simulink library "ddm"  (R2021b)
settings: Solver=VariableStepAuto  StartTime=0.0  StopTime=10.0  RelTol=1e-3
undefined symbols (not defined in the file or in its folder): ADDM_FrTMTqDev_X_Nm, ADDM_RrTMTqDev_X_Nm, ENUM_ADASACCSTA_ERROR, ENUM_ADASACCSTA_OFF, ENUM_ADASACCSTA_STANDBY, ENUM_ALLOWMOV_ALLOWREADY, ENUM_APS, ENUM_BRKSTA_ERROR, ENUM_BRKSTA_OFF, ENUM_BRKSTA_ON, ENUM_BRKSW_INVALID, ENUM_BRKSW_OFF, ENUM_BRKSW_ON, ENUM_CHGPREACTERRSTA_OBCPRE, ENUM_DCDCFAULTSTA_ANYFAULTLV1, ENUM_DCDCFAULTSTA_ANYFAULTLV2, ENUM_DRIVETRAIN_AWD, ENUM_DRIVETRAIN_FWD, ENUM_DRIVETRAIN_RWD, ENUM_EDUDRTSTA_NORMAL, ENUM_EPBSTA_APPLIED, ENUM_EPBSTA_RELEASED, ENUM_ESCAPSSta_APSUNAVAILABLE, ENUM_GEARACTUALPOSN_INVALID, ENUM_GEARACTUALPOSN_P, ENUM_HVBATTREADYPRE_READY, ENUM_MCUWARN_LV0, ENUM_MCUWARN_LV1, ENUM_MCUWARN_LV2, ENUM_MCUWARN_LV3, ENUM_MCUWARN_NOERROR, ENUM_OBCFAULTSTA_ANYFAULT, ENUM_PAS_R2F2, ENUM_PDFAULT_BATTPDFAIL, ENUM_PDFAULT_DCDCDISABLE, ENUM_PDFAULT_MCUDISABLE, ENUM_PDFAULT_MCUDISCHRG, ENUM_POWERSTA_OFF, ENUM_POWERSTA_ON, ENUM_POWERSTA_READY, ENUM_POWERSTA_STANDBY, ENUM_PRESSINDI_LOW, ENUM_PUFAULT_BATTUPFAIL, ENUM_PUFAULT_DCDCENABLEFAIL, ENUM_PUFAULT_PRECHRGCHKFAIL, ENUM_PUFAULT_SAFETYCHKFAIL, ENUM_PUSTATE_COMPLETED, ENUM_PWRSTASW_OFF, ENUM_PWRSTASW_OFFA, ENUM_PWRSTASW_OFFCHVCHRG, ENUM_PWRSTASW_OFFCLVCHRG, ENUM_PWRSTASW_ON, ENUM_PWRSTASW_ONHVCHRG, ENUM_PWRSTASW_READY, ENUM_PWRSTASW_STANDBY, ENUM_RAPSErrWarnSta_NORMAL, ENUM_RAPSErrWarnSta_RAPSERRLV1, ENUM_SHIFTCOMMAND_P, ENUM_SHIFTERERRSTA_PBUTTONFAILURE, ENUM_VEHMALFUNLV_2ND ... (+463)
libraries: hcu_lib x529, $bdroot x5, simulink x4
(part 12 of 25)

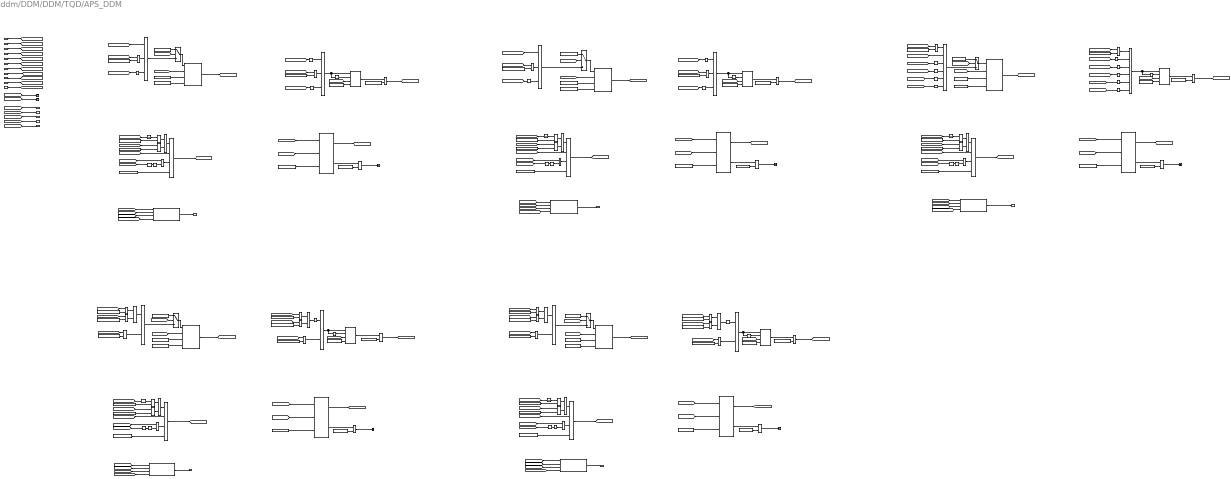
== system ddm/DDM/DDM/TQD/APS_DDM ==
  note: Release Condition After Decision
  note: Diagnostics and Fault Handling
  note: Diagnostics and Fault Handling
  note: Release Condition After Decision
  note: Release Condition After Decision
  note: Diagnostics and Fault Handling
  note: Diagnostics and Fault Handling
  note: Release Condition After Decision
  note: Release Condition After Decision
  note: Diagnostics and Fault Handling
  note: APS1 Signal Out of Range (APS1SigOoR)
  note: APS1 5V Out of Range (5vAPS1OoR)
  note: APS Correlation Error (APSCorrErr)
  note: APS2 Signal Out of Range (APS2SigOoR)
  note: APS2 5V Out of Range (5vAPS2OoR)
  VPMM_SysPwrSta_enum : Inport
  VINP_AccelPedal1Vol_V : Inport  Port=2
  VINP_AccelPedal2Vol_V : Inport  Port=3
  VDHP_EAPS12RangeSta_enum : Inport  Port=4
  VDHP_EAPCRBAD_flg : Inport  Port=5
  VINP_Pedal1Ref5V_V : Inport  Port=6
  VINP_Pedal2Ref5V_V : Inport  Port=7
  task_time_s : Inport  Port=8
  DTC_clear_request : Inport  Port=9
  VDHP_EAPS1BAD_flg : Inport  Port=10
  VDHP_EAPS2BAD_flg : Inport  Port=11
  Constant{1,7,10,14,17,23,27,34..39,41,48} (15 alike) : Constant  Value=ENUM_PWRSTASW_OFF
  Constant107 : Constant  Value=KDDM_APS2SigOoRPassTO_s
  Constant108 : Constant  Value=KDDM_APS2SigOoRPassTO_s
  Constant109 : Constant  Value=KDDM_5vAPS2OoRPassTO_s
  Constant{4,11,24,26,45} (5 alike) : Constant  Value=ENUM_PWRSTASW_STANDBY
  Constant{21,85,90,99,111} (5 alike) : Constant  Value=FALSE
  Constant112 : Constant  Value=KDDM_5vAPS2OoRDetTO_s
  Constant118 : Constant  Value=KDDM_5vAPS2OoRDTC_cnt
  Constant{6,12,31,46,53} (5 alike) : Constant  Value=KDDM_TQDDiagnosisOffSW_flg
  Constant{13,16,32,47,54} (5 alike) : Constant  Value=ZERO_INT
  Constant132 : Constant  Value=KDDM_APS1SigOoRDTC_cnt
  Constant15 : Constant  Value=KDDM_APS2SigOoRDTC_cnt
  Constant18 : Constant  Value=KDDM_5vAPS2OoRDTC_cnt
  Constant19 : Constant  Value=KDDM_5vAPS1OoRPassTO_s
  Constant2 : Constant  Value=KDDM_5vAPS1OoRHiLim_V
  Constant20 : Constant  Value=KDDM_5vAPS1OoRPassTO_s
  Constant22 : Constant  Value=KDDM_5vAPS1OoRDetTO_s
  Constant25 : Constant  Value=KDDM_5vAPS2OoRHiLim_V
  Constant28 : Constant  Value=KDDM_5vAPS2OoRHiLim_V
  Constant29 : Constant  Value=KDDM_5vAPS2OoRLoLim_V
  Constant3 : Constant  Value=KDDM_5vAPS1OoRLoLim_V
  Constant30 : Constant  Value=KDDM_5vAPS2OoRPassTO_s
  Constant33 : Constant  Value=KDDM_5vAPS2OoRLoLim_V
  Constant49 : Constant  Value=KDDM_APS1SigOoRDTC_cnt
  Constant5 : Constant  Value=KDDM_5vAPS1OoRDTC_cnt
  Constant50 : Constant  Value=KDDM_APS2SigOoRDTC_cnt
  Constant55 : Constant  Value=KDDM_APSCorrErrPassTO_s
  Constant57 : Constant  Value=KDDM_APSCorrErrDetTO_s
  Constant58 : Constant  Value=KDDM_APSCorrErrDTC_cnt
  Constant59 : Constant  Value=KDDM_APSCorrErrDTC_cnt
  Constant65 : Constant  Value=KDDM_5vAPS1OoRDTC_cnt
  Constant68 : Constant  Value=KDDM_APS2SigOoRDetTO_s
  Constant69 : Constant  Value=KDDM_APS1SigOoRPassTO_s
  Constant70 : Constant  Value=KDDM_APS1SigOoRPassTO_s
  Constant8 : Constant  Value=KDDM_5vAPS1OoRHiLim_V
  Constant86 : Constant  Value=KDDM_APS1SigOoRDetTO_s
  Constant9 : Constant  Value=KDDM_5vAPS1OoRLoLim_V
  Constant91 : Constant  Value=KDDM_APSCorrErrPassTO_s
  DTC_Couter{1..4,6} (5 alike) : hcu_lib/Basic_Blocks/DTC_Couter
  DTC_Info{,1..4} (5 alike) : hcu_lib/Basic_Blocks/DTC_Info
  Delay{1..5} (5 alike) : Delay  DelayLength=1
  Equal{1,3,6,13,15..16,19,21,26,47} (10 alike) : RelationalOperator  Operator=~=  OutDataTypeStr=boolean  RndMeth=Simplest
  Equal{4,10..12,18,23..25,39..40} (10 alike) : RelationalOperator  Operator===  OutDataTypeStr=boolean  RndMeth=Simplest
  Equal{2,7,14,20} (4 alike) : RelationalOperator  Operator=>  OutDataTypeStr=boolean  RndMeth=Simplest
  Equal{5,8,17,27} (4 alike) : RelationalOperator  Operator=<  OutDataTypeStr=boolean  RndMeth=Simplest
  Equal{9,28,55,65,70} (5 alike) : RelationalOperator  OutDataTypeStr=boolean  RndMeth=Simplest
  Logical Operator{1..2,14,17} (4 alike) : Logic  Operator=OR  AllPortsSameDT=off  OutDataTypeStr=boolean
  Logical Operator{3,7,10..12,19..20,22,29,34,37,39,41..42} (14 alike) : Logic  AllPortsSameDT=off  OutDataTypeStr=boolean
  Logical Operator{4,8,13,15..16,21,23..28,30,32,36,40,44..45,62,73,83,112} (22 alike) : Logic  Operator=NOT  AllPortsSameDT=off  OutDataTypeStr=boolean
  Logical Operator{6,9,18,38,43} (5 alike) : Logic  Operator=OR  Inputs=4  AllPortsSameDT=off  OutDataTypeStr=boolean
  Logical Operator{5,31,33,35} (4 alike) : Logic  Inputs=3  AllPortsSameDT=off  OutDataTypeStr=boolean
  Logical Operator49 : Logic  Inputs=6  AllPortsSameDT=off  OutDataTypeStr=boolean
  Logical Operator86 : Logic  Inputs=6  AllPortsSameDT=off  OutDataTypeStr=boolean
  NOT{1..5} (5 alike) : Logic  Operator=NOT  AllPortsSameDT=off  OutDataTypeStr=boolean
  Relational Operator{1..5} (5 alike) : RelationalOperator  Operator=>  OutDataTypeStr=boolean  RndMeth=Simplest
  Switch{1..4,6} (5 alike) : Switch  Criteria=u2 ~= 0
  Terminator{,1..6} (7 alike) : Terminator
  Test Detection Criteria{1..5} (5 alike) : hcu_lib/Basic_Blocks/Test Detection Criteria
  Timer{1,4..5,13,15} (5 alike) : hcu_lib/Basic_Blocks/Timer
  Unit Delay{1,3..6} (5 alike) : UnitDelay  SampleTime=-1  HasFrameUpgradeWarning=on
  VDDM_APS1SigOoRDTC_raw32 : Outport
  VDDM_APS2SigOoRDTC_raw32 : Outport  Port=2
  VDDM_APSCorrErrDTC_raw32 : Outport  Port=3
  VDDM_5vAPS1OoRDTC_raw32 : Outport  Port=4
  VDDM_5vAPS2OoRDTC_raw32 : Outport  Port=5
  VDDM_5vAPS1OoRCFS_flg : Outport  Port=6
  VDDM_5vAPS2OoRCFS_flg : Outport  Port=7
  VDDM_APS1SigOoRCFS_flg : Outport  Port=8
  VDDM_APS2SigOoRCFS_flg : Outport  Port=9
  VDDM_APSCorrErrCFS_flg : Outport  Port=10
  wires:
  Logical Operator44/1 -> Logical Operator49/6
  Logical Operator27/1 -> Logical Operator49/5
  Logical Operator26/1 -> Logical Operator49/4
  Logical Operator25/1 -> Logical Operator49/3
  Logical Operator24/1 -> Logical Operator86/6
  Logical Operator21/1 -> Logical Operator86/5
  Logical Operator16/1 -> Logical Operator86/4
  Logical Operator15/1 -> Logical Operator86/3
  Logical Operator13/1 -> Logical Operator35/1
  [VDDM_APS1SigOoRCFS_flg] -> Logical Operator27/1
  [VDDM_APS2SigOoRCFS_flg] -> Logical Operator44/1
  [VDDM_5vAPS2OoRCFS_flg] -> Logical Operator26/1
  [VDDM_5vAPS1OoRCFS_flg] -> Logical Operator25/1
  Equal26/1 -> Logical Operator49/1
  Constant41/1 -> Equal26/2
  [VPMM_SysPwrSta_enum] -> Equal26/1
  [VDDM_APS2SigOoRCFS_flg] -> Logical Operator24/1
  [VDDM_APS1SigOoRCFS_flg] -> Logical Operator21/1
  [VDDM_5vAPS2OoRCFS_flg] -> Logical Operator16/1
  [VDDM_5vAPS1OoRCFS_flg] -> Logical Operator15/1
  Equal21/1 -> Logical Operator86/1
  [VPMM_SysPwrSta_enum] -> Equal21/1
  Constant39/1 -> Equal21/2
  [VPMM_SysPwrSta_enum] -> Equal16/1
  Constant38/1 -> Equal16/2
  [VPMM_SysPwrSta_enum] -> Equal3/1
  Constant10/1 -> Equal3/2
  [VPMM_SysPwrSta_enum] -> Equal15/1
  Constant37/1 -> Equal15/2
  [VPMM_SysPwrSta_enum] -> Equal47/1
  Constant36/1 -> Equal47/2
  [VDDM_APSCorrErrCFS_flg] -> VDDM_APSCorrErrCFS_flg/1
  [VDDM_APS2SigOoRCFS_flg] -> VDDM_APS2SigOoRCFS_flg/1
  [VDDM_APS1SigOoRCFS_flg] -> VDDM_APS1SigOoRCFS_flg/1
  [VDDM_5vAPS2OoRCFS_flg] -> VDDM_5vAPS2OoRCFS_flg/1
  [VDDM_5vAPS1OoRCFS_flg] -> VDDM_5vAPS1OoRCFS_flg/1
  Logical Operator23/1 -> Logical Operator22/1
  Equal27/1 -> Logical Operator14/2
  Constant29/1 -> Equal27/2
  Equal20/1 -> Logical Operator14/1
  [VINP_Pedal2Ref5V_V] -> Equal20/1
  Logical Operator14/1 -> Logical Operator23/1
  Constant28/1 -> Equal20/2
  Constant27/1 -> Equal19/2
  [VPMM_SysPwrSta_enum] -> Equal19/1
  [VINP_Pedal2Ref5V_V] -> Equal27/1
  Equal19/1 -> Logical Operator22/2
  Equal13/1 -> Logical Operator20/2
  [VINP_Pedal2Ref5V_V] -> Equal17/1
  [VPMM_SysPwrSta_enum] -> Equal13/1
  Constant23/1 -> Equal13/2
  Constant25/1 -> Equal14/2
  Logical Operator17/1 -> Logical Operator20/1
  [VINP_Pedal2Ref5V_V] -> Equal14/1
  Equal14/1 -> Logical Operator17/1
  Constant33/1 -> Equal17/2
  Equal17/1 -> Logical Operator17/2
  [VDDM_5vAPS2OoRDet_flg] -> DTC_Couter4/1
  [VDDM_5vAPS2OoRCFSRls_flg] -> DTC_Couter4/2
  [VPMM_SysPwrSta_enum] -> Unit Delay1/1
  Constant16/1 -> Relational Operator5/2
  [VDDM_5vAPS2OoRCFS_flg] -> Delay5/1
  Logical Operator10/1 -> Logical Operator9/1
  Equal11/1 -> Logical Operator10/1
  Constant6/1 -> Logical Operator9/4
  Logical Operator9/1 -> [VDDM_5vAPS2OoRCFSRls_flg]  "VDDM_5vAPS2OoRCFSRls_flg"
  Delay5/1 -> NOT5/1
  NOT5/1 -> Logical Operator11/2
  [DTC_clear_request] -> Logical Operator9/2
  Constant4/1 -> Equal10/2
  Constant18/1 -> DTC_Couter4/3
  Equal10/1 -> Logical Operator10/2
  DTC_Couter4/2 -> Relational Operator5/1  "VDDM_5vAPS2OoRDTC_cnt"
  [VPMM_SysPwrSta_enum] -> Equal10/1
  Logical Operator11/1 -> Logical Operator9/3
  Constant17/1 -> Equal11/2
  Unit Delay1/1 -> Equal11/1
  Relational Operator5/1 -> Terminator4/1  "VDDM_5vAPS2OoRDFS_flg"
  [VDDM_5vAPS2OoRPass_flg] -> Logical Operator11/1
  DTC_Couter4/1 -> [VDDM_5vAPS2OoRCFS_flg]  "VDDM_5vAPS2OoRCFS_flg"
  Logical Operator8/1 -> Logical Operator7/1
  Equal6/1 -> Logical Operator7/2
  [VINP_Pedal1Ref5V_V] -> Equal8/1
  [VPMM_SysPwrSta_enum] -> Equal6/1
  Constant1/1 -> Equal6/2
  Constant2/1 -> Equal7/2
  Logical Operator1/1 -> Logical Operator8/1
  [VINP_Pedal1Ref5V_V] -> Equal7/1
  Equal7/1 -> Logical Operator1/1
  Constant3/1 -> Equal8/2
  Equal8/1 -> Logical Operator1/2
  Constant65/1 -> DTC_Couter3/3
  [VDDM_5vAPS1OoRDet_flg] -> DTC_Couter3/1
  Equal12/1 -> Logical Operator19/2
  Relational Operator4/1 -> Terminator3/1  "VDDM_5vAPS1OoRDFS_flg"
  [VDDM_5vAPS1OoRCFSRls_flg] -> DTC_Couter3/2
  [VDDM_5vAPS1OoRPass_flg] -> Logical Operator34/1
  Logical Operator18/1 -> [VDDM_5vAPS1OoRCFSRls_flg]  "VDDM_5vAPS1OoRCFSRls_flg"
  Constant31/1 -> Logical Operator18/4
  Logical Operator19/1 -> Logical Operator18/1
  [VPMM_SysPwrSta_enum] -> Unit Delay5/1
  Constant24/1 -> Equal12/2
  [DTC_clear_request] -> Logical Operator18/2
  NOT4/1 -> Logical Operator34/2
  Delay4/1 -> NOT4/1
  DTC_Couter3/1 -> [VDDM_5vAPS1OoRCFS_flg]  "VDDM_5vAPS1OoRCFS_flg"
  Equal18/1 -> Logical Operator19/1
  Unit Delay5/1 -> Equal18/1
  Constant35/1 -> Equal18/2
  Constant32/1 -> Relational Operator4/2
  DTC_Couter3/2 -> Relational Operator4/1  "VDDM_5vAPS1OoRDTC_cnt"
  Logical Operator34/1 -> Logical Operator18/3
  [VPMM_SysPwrSta_enum] -> Equal12/1
  [VDDM_5vAPS1OoRCFS_flg] -> Delay4/1
  Constant7/1 -> Equal1/2
  [VPMM_SysPwrSta_enum] -> Equal1/1
  Unit Delay4/1 -> Equal39/1
  Constant54/1 -> Relational Operator3/2
  Constant34/1 -> Equal39/2
  DTC_Couter2/2 -> Relational Operator3/1  "VDDM_APSCorrErrDTC_cnt"
  Logical Operator42/1 -> Logical Operator43/3
  [VDDM_APSCorrErrCFS_flg] -> Delay3/1
  Logical Operator43/1 -> [VDDM_APSCorrErrCFSRls_flg]  "VDDM_APSCorrErrCFSRls_flg"
  [VPMM_SysPwrSta_enum] -> Equal40/1
  Relational Operator3/1 -> Terminator2/1  "VDDM_APSCorrErrDFS_flg"
  Equal40/1 -> Logical Operator37/2
  Constant59/1 -> DTC_Couter2/3
  Equal39/1 -> Logical Operator37/1
  DTC_Couter2/1 -> [VDDM_APSCorrErrCFS_flg]  "VDDM_APSCorrErrCFS_flg"
  [VDDM_APSCorrErrPass_flg] -> Logical Operator42/1
  [VDDM_APSCorrErrDet_flg] -> DTC_Couter2/1
  Logical Operator37/1 -> Logical Operator43/1
  Constant53/1 -> Logical Operator43/4
  Delay3/1 -> NOT3/1
  NOT3/1 -> Logical Operator42/2
  [DTC_clear_request] -> Logical Operator43/2
  Constant26/1 -> Equal40/2
  [VPMM_SysPwrSta_enum] -> Unit Delay4/1
  [VDDM_APSCorrErrCFSRls_flg] -> DTC_Couter2/2
  [VDDM_APS2SigOoRCFSRls_flg] -> Switch1/2
  [VDHP_EAPS2BAD_flg] -> Logical Operator13/1
  [VDDM_5vAPS2OoRCFS_flg] -> Logical Operator32/1
  Equal16/1 -> Logical Operator35/2
  Logical Operator32/1 -> Logical Operator35/3
  Constant50/1 -> DTC_Couter1/3
  [VDDM_APS2SigOoRDet_flg] -> DTC_Couter1/1
  Equal4/1 -> Logical Operator12/2
  Relational Operator1/1 -> Terminator1/1  "VDDM_APS2SigOoRDFS_flg"
  [VDDM_APS2SigOoRCFSRls_flg] -> DTC_Couter1/2
  [VDDM_APS2SigOoRPass_flg] -> Logical Operator29/1
  Logical Operator6/1 -> [VDDM_APS2SigOoRCFSRls_flg]  "VDDM_APS2SigOoRCFSRls_flg"
  Constant12/1 -> Logical Operator6/4
  Logical Operator12/1 -> Logical Operator6/1
  [VPMM_SysPwrSta_enum] -> Unit Delay3/1
  Constant11/1 -> Equal4/2
  [DTC_clear_request] -> Logical Operator6/2
  NOT2/1 -> Logical Operator29/2
  Delay2/1 -> NOT2/1
  DTC_Couter1/1 -> [VDDM_APS2SigOoRCFS_flg]  "VDDM_APS2SigOoRCFS_flg"
  Equal25/1 -> Logical Operator12/1
  Unit Delay3/1 -> Equal25/1
  Constant14/1 -> Equal25/2
  Constant13/1 -> Relational Operator1/2
  DTC_Couter1/2 -> Relational Operator1/1  "VDDM_APS2SigOoRDTC_cnt"
  Logical Operator29/1 -> Logical Operator6/3
  [VPMM_SysPwrSta_enum] -> Equal4/1
  [VDDM_APS2SigOoRCFS_flg] -> Delay2/1
  Logical Operator5/1 -> Switch1/3
  Logical Operator4/1 -> Logical Operator5/3
  Equal3/1 -> Logical Operator5/2
  [VDDM_5vAPS2OoRCFS_flg] -> Logical Operator4/1
  [VDHP_EAPS2BAD_flg] -> Logical Operator5/1
  Delay1/1 -> NOT1/1
  [VDDM_APS1SigOoRCFS_flg] -> Delay1/1
  Constant46/1 -> Logical Operator38/4
  [DTC_clear_request] -> Logical Operator38/2
  NOT1/1 -> Logical Operator41/2
  Constant45/1 -> Equal23/2
  Logical Operator39/1 -> Logical Operator38/1
  [VPMM_SysPwrSta_enum] -> Unit Delay6/1
  Relational Operator2/1 -> Terminator/1  "VDDM_APS1SigOoRDFS_flg"
  Equal23/1 -> Logical Operator39/2
  Constant48/1 -> Equal24/2
  Unit Delay6/1 -> Equal24/1
  [VPMM_SysPwrSta_enum] -> Equal23/1
  Equal24/1 -> Logical Operator39/1
  [VDDM_APS1SigOoRPass_flg] -> Logical Operator41/1
  Logical Operator41/1 -> Logical Operator38/3
  Constant49/1 -> DTC_Couter6/3
  DTC_Couter6/1 -> [VDDM_APS1SigOoRCFS_flg]  "VDDM_APS1SigOoRCFS_flg"
  Logical Operator38/1 -> [VDDM_APS1SigOoRCFSRls_flg]  "VDDM_APS1SigOoRCFSRls_flg"
  [VDDM_APS1SigOoRCFSRls_flg] -> DTC_Couter6/2
  DTC_Couter6/2 -> Relational Operator2/1  "VDDM_APS1SigOoRDTC_cnt"
  [VDDM_APS1SigOoRDet_flg] -> DTC_Couter6/1
  Constant47/1 -> Relational Operator2/2
  Logical Operator36/1 -> Logical Operator33/1
  [VDHP_EAPS1BAD_flg] -> Logical Operator36/1
  [VDDM_5vAPS1OoRCFS_flg] -> Logical Operator30/1
  Equal15/1 -> Logical Operator33/2
  Logical Operator30/1 -> Logical Operator33/3
  [VDDM_APSCorrErrPass_flg] -> DTC_Info2/2
  [VDDM_APSCorrErrDet_flg] -> DTC_Info2/1
  [VDDM_APS2SigOoRPass_flg] -> DTC_Info1/2
  [VDDM_APS2SigOoRDet_flg] -> DTC_Info1/1
  [VDDM_APS1SigOoRDet_flg] -> DTC_Info/1
  DTC_clear_request/1 -> [DTC_clear_request]
  task_time_s/1 -> [task_time_s]
  Logical Operator28/1 -> Logical Operator31/3
  Equal47/1 -> Logical Operator31/2
  [VDDM_5vAPS1OoRCFS_flg] -> Logical Operator28/1
  [VDHP_EAPS1BAD_flg] -> Logical Operator31/1
  Logical Operator73/1 -> Timer1/2
  Constant69/1 -> Equal28/2
  Timer1/1 -> Equal28/1
  Constant70/1 -> Timer1/4
  [task_time_s] -> Timer1/3
  Constant57/1 -> Test Detection Criteria1/4
  [task_time_s] -> Timer13/3
  Timer13/1 -> Equal55/1
  Logical Operator83/1 -> Timer13/2
  Test Detection Criteria1/1 -> [VDDM_APSCorrErrDet_flg]  "VDDM_APSCorrErrDet_flg"
  Constant91/1 -> Equal55/2
  [task_time_s] -> Test Detection Criteria1/2
  Constant55/1 -> Timer13/4
  Equal28/1 -> [VDDM_APS1SigOoRPass_flg]  "VDDM_APS1SigOoRPass_flg"
  Logical Operator35/1 -> Logical Operator112/1, Timer15/1
  Test Detection Criteria4/1 -> [VDDM_APS2SigOoRDet_flg]  "VDDM_APS2SigOoRDet_flg"
  Constant107/1 -> Equal65/2
  Constant108/1 -> Timer15/4
  Logical Operator112/1 -> Timer15/2
  Timer15/1 -> Equal65/1
  Equal65/1 -> [VDDM_APS2SigOoRPass_flg]  "VDDM_APS2SigOoRPass_flg"
  [task_time_s] -> Timer15/3
  Equal55/1 -> [VDDM_APSCorrErrPass_flg]  "VDDM_APSCorrErrPass_flg"
  Logical Operator49/1 -> Logical Operator83/1, Timer13/1
  [task_time_s] -> Test Detection Criteria3/2
  Constant86/1 -> Test Detection Criteria3/4
  Constant132/1 -> Test Detection Criteria3/3
  Test Detection Criteria3/1 -> [VDDM_APS1SigOoRDet_flg]  "VDDM_APS1SigOoRDet_flg"
  [VDDM_APS1SigOoRCFS_flg] -> DTC_Info/3
  [VDDM_APS1SigOoRPass_flg] -> DTC_Info/2
  DTC_Info/1 -> VDDM_APS1SigOoRDTC_raw32/1  "VDDM_APS1SigOoRDTC_raw32"
  Logical Operator33/1 -> Timer1/1, Logical Operator73/1
  [task_time_s] -> Test Detection Criteria4/2
  Constant15/1 -> Test Detection Criteria4/3
  Constant68/1 -> Test Detection Criteria4/4
  [VDDM_APS2SigOoRCFS_flg] -> DTC_Info1/3
  DTC_Info1/1 -> VDDM_APS2SigOoRDTC_raw32/1  "VDDM_APS2SigOoRDTC_raw32"
  VPMM_SysPwrSta_enum/1 -> [VPMM_SysPwrSta_enum]
  VINP_AccelPedal1Vol_V/1 -> [VINP_AccelPedal1Vol_V]
  VINP_AccelPedal2Vol_V/1 -> [VINP_AccelPedal2Vol_V]
  Constant58/1 -> Test Detection Criteria1/3
  [VDDM_APSCorrErrCFS_flg] -> DTC_Info2/3
  DTC_Info2/1 -> VDDM_APSCorrErrDTC_raw32/1  "VDDM_APSCorrErrDTC_raw32"
  VDHP_EAPS12RangeSta_enum/1 -> [VDHP_EAPS12RangeSta_enum]
  VDHP_EAPCRBAD_flg/1 -> [VDHP_EAPCRBAD_flg]
  [DTC_clear_request] -> DTC_Info/4
  [DTC_clear_request] -> DTC_Info1/4
  [DTC_clear_request] -> DTC_Info2/4
  [VDDM_APS1SigOoRCFSRls_flg] -> Switch6/2
  Switch6/1 -> Test Detection Criteria3/1
  Logical Operator31/1 -> Switch6/3
  Constant85/1 -> Switch6/1
  Switch1/1 -> Test Detection Criteria4/1
  Constant90/1 -> Switch1/1
  [VDDM_APSCorrErrCFSRls_flg] -> Switch2/2
  Switch2/1 -> Test Detection Criteria1/1
  Logical Operator86/1 -> Switch2/3
  Constant99/1 -> Switch2/1
  VINP_Pedal1Ref5V_V/1 -> [VINP_Pedal1Ref5V_V]
  VINP_Pedal2Ref5V_V/1 -> [VINP_Pedal2Ref5V_V]
  [VDDM_5vAPS1OoRCFS_flg] -> DTC_Info3/3
  [VDDM_5vAPS1OoRDet_flg] -> DTC_Info3/1
  Constant22/1 -> Test Detection Criteria2/4
  Timer4/1 -> Equal9/1
  Constant20/1 -> Timer4/4
  Logical Operator40/1 -> Timer4/2
  Test Detection Criteria2/1 -> [VDDM_5vAPS1OoRDet_flg]  "VDDM_5vAPS1OoRDet_flg"
  [VDDM_5vAPS1OoRCFSRls_flg] -> Switch3/2
  Constant19/1 -> Equal9/2
  [VDDM_5vAPS1OoRPass_flg] -> DTC_Info3/2
  Constant5/1 -> Test Detection Criteria2/3
  [task_time_s] -> Test Detection Criteria2/2
  [DTC_clear_request] -> DTC_Info3/4
  DTC_Info3/1 -> VDDM_5vAPS1OoRDTC_raw32/1  "VDDM_5vAPS1PwrErrDTC_raw32"
  Switch3/1 -> Test Detection Criteria2/1
  [task_time_s] -> Timer4/3
  Logical Operator7/1 -> Timer4/1, Logical Operator40/1
  Constant21/1 -> Switch3/1
  Equal9/1 -> [VDDM_5vAPS1OoRPass_flg]  "VDDM_5vAPS1OoRPass_flg"
  Equal2/1 -> Logical Operator2/1
  Equal5/1 -> Logical Operator2/2
  Logical Operator2/1 -> Logical Operator3/1
  Constant8/1 -> Equal2/2
  Constant9/1 -> Equal5/2
  Logical Operator3/1 -> Switch3/3
  [VINP_Pedal1Ref5V_V] -> Equal2/1
  [VINP_Pedal1Ref5V_V] -> Equal5/1
  VDHP_EAPS2BAD_flg/1 -> [VDHP_EAPS2BAD_flg]
  Switch4/1 -> Test Detection Criteria5/1
  [VDDM_5vAPS2OoRDet_flg] -> DTC_Info4/1
  Logical Operator22/1 -> Timer5/1, Logical Operator62/1
  Constant112/1 -> Test Detection Criteria5/4
  [VDDM_5vAPS2OoRCFSRls_flg] -> Switch4/2
  Constant30/1 -> Equal70/2
  [VDDM_5vAPS2OoRPass_flg] -> DTC_Info4/2
  [task_time_s] -> Test Detection Criteria5/2
  Constant118/1 -> Test Detection Criteria5/3
  [task_time_s] -> Timer5/3
  [DTC_clear_request] -> DTC_Info4/4
  Constant111/1 -> Switch4/1
  Constant109/1 -> Timer5/4
  [VDDM_5vAPS2OoRCFS_flg] -> DTC_Info4/3
  Equal70/1 -> [VDDM_5vAPS2OoRPass_flg]  "VDDM_5vAPS2OoRPass_flg"
  DTC_Info4/1 -> VDDM_5vAPS2OoRDTC_raw32/1  "VDDM_5vAPS2PwrErrDTC_raw32"
  Logical Operator62/1 -> Timer5/2
  Test Detection Criteria5/1 -> [VDDM_5vAPS2OoRDet_flg]  "VDDM_5vAPS2OoRDet_flg"
  Timer5/1 -> Equal70/1
  Logical Operator20/1 -> Switch4/3
  VDHP_EAPS1BAD_flg/1 -> [VDHP_EAPS1BAD_flg]
  Equal1/1 -> Logical Operator3/2
  [VINP_AccelPedal1Vol_V] -> Terminator5/1
  [VINP_AccelPedal2Vol_V] -> Terminator6/1
  [VDHP_EAPCRBAD_flg] -> Logical Operator86/2
  [VDHP_EAPCRBAD_flg] -> Logical Operator45/1
  Logical Operator45/1 -> Logical Operator49/2

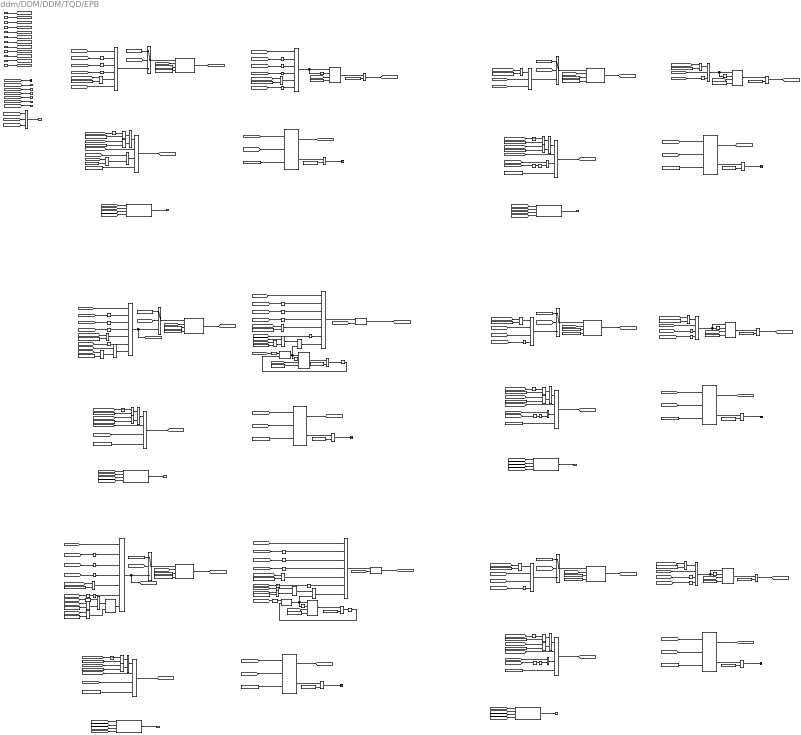
== system ddm/DDM/DDM/TQD/EPB ==
  note: EPB Release Response Timeout (EPBUnlockTO)
  note: EPB Apply Response Timeout (EPBLockTO)
  note: Release Condition After Decision
  note: Release Condition After Decision
  note: EPB1 CheckSum Error (EPB1CSErr)
  note: EPB1 Rolling Count Error (EPB1RCErr)
  note: EPB1 Lost Comm (EPB1NoCom)
  note: Release Condition After Decision
  note: Diagnostics and Fault Handling
  note: Diagnostics and Fault Handling
  note: Diagnostics and Fault Handling
  note: EPB Signal Error (EPBSigErr)
  note: Release Condition After Decision
  note: Diagnostics and Fault Handling
  note: Release Condition After Decision
  note: Diagnostics and Fault Handling
  note: Release Condition After Decision
  note: Diagnostics and Fault Handling
  NO_CAN1_BUS_OFF : Inport
  VTQD_GearActualPosn_enum : Inport  Port=2
  VINP_EPBErrSta_enum : Inport  Port=3
  VPMM_SysPwrSta_enum : Inport  Port=4
  VTQD_ActParkRequest_flg : Inport  Port=5
  VINP_EPBSta_enum : Inport  Port=6
  VINP_ShifterHandleCmd_enum : Inport  Port=7
  task_time_s : Inport  Port=8
  DTC_clear_request : Inport  Port=9
  VDDM_EPB1NoCom_flg : Inport  Port=10
  VDDM_EPB1RCErr_flg : Inport  Port=11
  VDDM_EPB1CSErr_flg : Inport  Port=12
  AND{,1..5} (6 alike) : Logic  AllPortsSameDT=off  OutDataTypeStr=boolean
  Constant{1,4,8,14,19,26,28,30,32,37,51,71,77,81,83..85,99} (18 alike) : Constant  Value=ENUM_PWRSTASW_OFF
  Constant10 : Constant  Value=ENUM_EPBSTA_APPLIED
  Constant{5,23,48,60,88,101} (6 alike) : Constant  Value=KDDM_TQDDiagnosisOffSW_flg
  Constant{17,21,54,76,94,102} (6 alike) : Constant  Value=ZERO_INT
  Constant11 : Constant  Value=ENUM_EPBSTA_RELEASED
  Constant12 : Constant  Value=KDDM_EPBLockTODTC_cnt
  Constant{13,18,25,27,29,31} (6 alike) : Constant  Value=ENUM_PWRSTASW_STANDBY
  Constant15 : Constant  Value=KDDM_EPBUnlockTOPassTO_s
  Constant16 : Constant  Value=KDDM_EPBUnlockTODTC_cnt
  Constant{2,35,55,65,72,96} (6 alike) : Constant  Value=FALSE
  Constant20 : Constant  Value=KDDM_EPBLockTODTC_cnt
  Constant22 : Constant  Value=KDDM_EPBLockTODetTO_s
  Constant24 : Constant  Value=KDDM_EPB1RCErrDTC_cnt
  Constant3 : Constant  Value=ENUM_EPBSTA_RELEASED
  Constant33 : Constant  Value=KDDM_EPBLockTOPassTO_s
  Constant34 : Constant  Value=KDDM_EPBLockTOPassTO_s
  Constant36 : Constant  Value=KDDM_EPBUnlockTODTC_cnt
  Constant38 : Constant  Value=KDDM_EPBUnlockTODetTO_s
  Constant50 : Constant  Value=ENUM_EPBSTA_APPLIED
  Constant56 : Constant  Value=KDDM_EPB1RCErrDTC_cnt
  Constant57 : Constant  Value=KDDM_EPB1RCErrPassTO_s
  Constant59 : Constant  Value=KDDM_EPB1CSErrDTC_cnt
  Constant6 : Constant  Value=KDDM_EPBUnlockTOPassTO_s
  Constant62 : Constant  Value=KDDM_EPB1NoComDTC_cnt
  Constant64 : Constant  Value=KDDM_EPB1RCErrDetTO_s
  Constant66 : Constant  Value=KDDM_EPB1NoComDTC_cnt
  Constant67 : Constant  Value=KDDM_EPB1NoComPassTO_s
  Constant69 : Constant  Value=KDDM_EPB1NoComDetTO_s
  Constant7 : Constant  Value=ENUM_EPBSTA_RELEASED
  Constant70 : Constant  Value=KDDM_EPB1RCErrPassTO_s
  Constant73 : Constant  Value=KDDM_EPB1CSErrDTC_cnt
  Constant74 : Constant  Value=KDDM_EPB1CSErrPassTO_s
  Constant75 : Constant  Value=KDDM_EPB1CSErrDetTO_s
  Constant78 : Constant  Value=KDDM_EPB1CSErrPassTO_s
  Constant79 : Constant  Value=KDDM_EPB1NoComPassTO_s
  Constant86 : Constant  Value=ONE_INT
  Constant87 : Constant  Value=KDDM_EPBSigErrPassTO_s
  Constant89 : Constant  Value=KDDM_EPBSigErrDTC_cnt
  Constant95 : Constant  Value=KDDM_EPBSigErrPassTO_s
  Constant97 : Constant  Value=KDDM_EPBSigErrDTC_cnt
  Constant98 : Constant  Value=KDDM_EPBSigErrDetTO_s
  DTC_Couter{1,3..7} (6 alike) : hcu_lib/Basic_Blocks/DTC_Couter
  DTC_Info{,1..5} (6 alike) : hcu_lib/Basic_Blocks/DTC_Info
  Delay{,1..4} (5 alike) : Delay  DelayLength=1
  Detect Decrease : simulink/Logic and Bit Operations/Detect Decrease  vinit=0.0  OutDataTypeStr=boolean
  Detect Decrease1 : simulink/Logic and Bit Operations/Detect Decrease  vinit=0.0  OutDataTypeStr=boolean
  Detect Increase : simulink/Logic and Bit Operations/Detect Increase  vinit=0.0  OutDataTypeStr=boolean
  Equal{1,3,5,9,11,27,29,37..38,41..42,45,47,53} (14 alike) : RelationalOperator  Operator=~=  OutDataTypeStr=boolean  RndMeth=Simplest
  Equal{2,4,6,8,10,12..21,54} (16 alike) : RelationalOperator  Operator===  OutDataTypeStr=boolean  RndMeth=Simplest
  Equal{7,22,36,39..40,52} (6 alike) : RelationalOperator  OutDataTypeStr=boolean  RndMeth=Simplest
  Logical Operator : Logic  Operator=OR  Inputs=3  AllPortsSameDT=off  OutDataTypeStr=boolean
  Logical Operator{1,23,52,58,74,79} (6 alike) : Logic  Operator=OR  Inputs=4  AllPortsSameDT=off  OutDataTypeStr=boolean
  Logical Operator{7,9..10,13,17..18,70..71,76,80} (10 alike) : Logic  AllPortsSameDT=off  OutDataTypeStr=boolean
  Logical Operator{5..6,8,11..12,14..16,20,28,30,34..36,38..39,42..44,53..54,56..57,59,62,64,66,68,73,82,88..91,93..95} (37 alike) : Logic  Operator=NOT  AllPortsSameDT=off  OutDataTypeStr=boolean
  Logical Operator{2..3,19,31} (4 alike) : Logic  Inputs=7  AllPortsSameDT=off  OutDataTypeStr=boolean
  Logical Operator{60,63,67,69} (4 alike) : Logic  Inputs=4  AllPortsSameDT=off  OutDataTypeStr=boolean
  Logical Operator65 : Logic  Inputs=3  AllPortsSameDT=off  OutDataTypeStr=boolean
  Logical Operator72 : Logic  Inputs=3  AllPortsSameDT=off  OutDataTypeStr=boolean
  Logical Operator86 : Logic  Inputs=6  AllPortsSameDT=off  OutDataTypeStr=boolean
  Logical Operator92 : Logic  Inputs=6  AllPortsSameDT=off  OutDataTypeStr=boolean
  NOT1 : Logic  Operator=NOT  AllPortsSameDT=off  OutDataTypeStr=boolean
  NOT2 : Logic  Operator=NOT  AllPortsSameDT=off  OutDataTypeStr=boolean
  NOT3 : Logic  Operator=NOT  AllPortsSameDT=off  OutDataTypeStr=boolean
  Relational Operator{1..6} (6 alike) : RelationalOperator  Operator=>  OutDataTypeStr=boolean  RndMeth=Simplest
  SR_Latch{,1..4} (5 alike) : hcu_lib/Basic_Blocks/SR_Latch
  Switch{1..6} (6 alike) : Switch  Criteria=u2 ~= 0
  Terminator{,1..6} (7 alike) : Terminator
  Test Detection Criteria{1..6} (6 alike) : hcu_lib/Basic_Blocks/Test Detection Criteria
  Timer{1..2,4..7} (6 alike) : hcu_lib/Basic_Blocks/Timer
  Unit Delay{1..8} (8 alike) : UnitDelay  SampleTime=-1  HasFrameUpgradeWarning=on
  VDDM_EPBLockTODTC_raw32 : Outport
  VDDM_EPBUnlockTODTC_raw32 : Outport  Port=2
  VDDM_EPBLockTOCFS_flg : Outport  Port=3
  VDDM_EPBUnlockTOCFS_flg : Outport  Port=4
  VDDM_EPB1NoComDTC_raw32 : Outport  Port=5
  VDDM_EPB1RCErrDTC_raw32 : Outport  Port=6
  VDDM_EPB1CSErrDTC_raw32 : Outport  Port=7
  VDDM_EPBSigErrDTC_raw32 : Outport  Port=8
  VDDM_EPBSigErrCFS_flg : Outport  Port=9
  VDDM_EPB1NoComCFS_flg : Outport  Port=10
  VDDM_EPB1RCErrCFS_flg : Outport  Port=11
  VDDM_EPB1CSErrCFS_flg : Outport  Port=12
  VDDM_EPB1Err_flg : Outport  Port=13
  wires:
  Logical Operator43/1 -> Logical Operator19/3
  [VDDM_EPB1CSErrCFS_flg] -> Logical Operator44/1
  Logical Operator44/1 -> Logical Operator19/4
  Logical Operator42/1 -> Logical Operator19/2
  [VDDM_EPB1RCErrCFS_flg] -> Logical Operator43/1
  [VDDM_EPB1NoComCFS_flg] -> Logical Operator42/1
  [VDDM_EPB1RCErrCFS_flg] -> Logical Operator35/1
  [VDDM_EPB1NoComCFS_flg] -> Logical Operator12/1
  Logical Operator35/1 -> Logical Operator3/3
  Logical Operator12/1 -> Logical Operator3/2
  Logical Operator36/1 -> Logical Operator3/4
  [VDDM_EPB1CSErrCFS_flg] -> Logical Operator36/1
  DTC_clear_request/1 -> [DTC_clear_request]
  task_time_s/1 -> [task_time_s]
  VINP_ShifterHandleCmd_enum/1 -> [VINP_ShifterHandleCmd_enum]
  VINP_EPBSta_enum/1 -> [VINP_EPBSta_enum]
  VTQD_ActParkRequest_flg/1 -> [VTQD_ActParkRequest_flg]
  VPMM_SysPwrSta_enum/1 -> [VPMM_SysPwrSta_enum]
  VINP_EPBErrSta_enum/1 -> [VINP_EPBErrSta_enum]
  VTQD_GearActualPosn_enum/1 -> [VTQD_GearActualPosn_enum]
  NO_CAN1_BUS_OFF/1 -> [NO_CAN1_BUS_OFF]
  [VINP_EPBSta_enum] -> Equal5/1
  Equal5/1 -> AND2/2
  Constant11/1 -> Equal5/2
  [VTQD_ActParkRequest_flg] -> AND/1
  Equal27/1 -> AND/2
  Constant50/1 -> Equal27/2
  [VINP_EPBSta_enum] -> Equal27/1
  Logical Operator19/1 -> [VDDM_EPBUnlockTOTestFail_flg], Switch1/3
  Equal9/1 -> Logical Operator19/5
  [NO_CAN1_BUS_OFF] -> Logical Operator19/1
  [VDDM_EPBLockTOCFS_flg] -> Unit Delay3/1
  Unit Delay3/1 -> Logical Operator28/1
  Logical Operator28/1 -> Logical Operator19/6
  AND/1 -> Logical Operator3/7
  [VDDM_EPBUnlockTOCFS_flg] -> Logical Operator30/1
  Logical Operator30/1 -> Logical Operator3/6
  [VDDM_EPBUnlockTOPass_flg] -> DTC_Info1/2
  [task_time_s] -> Test Detection Criteria2/2
  Constant35/1 -> Switch1/1
  Test Detection Criteria2/1 -> [VDDM_EPBUnlockTODet_flg]  "VDDM_EPBUnlockTODet_flg"
  [VDDM_EPBUnlockTODFSRls_flg] -> Switch1/2
  Constant38/1 -> Test Detection Criteria2/4
  [DTC_clear_request] -> DTC_Info1/4
  [VDDM_EPBUnlockTOCFS_flg] -> DTC_Info1/3
  Constant36/1 -> Test Detection Criteria2/3
  Switch1/1 -> Test Detection Criteria2/1
  DTC_Info1/1 -> VDDM_EPBUnlockTODTC_raw32/1  "VDDM_EPBUnlockTODTC_raw32"
  [VDDM_EPBUnlockTODet_flg] -> DTC_Info1/1
  [NO_CAN1_BUS_OFF] -> Logical Operator3/1
  Equal1/1 -> Logical Operator3/5
  [DTC_clear_request] -> DTC_Info/4
  [VDDM_EPBLockTOCFSRls_flg] -> Switch6/2
  Test Detection Criteria1/1 -> [VDDM_EPBLockTODet_flg]  "VDDM_EPBLockTODet_flg"
  DTC_Info/1 -> VDDM_EPBLockTODTC_raw32/1  "VDDM_EPBLockTODTC_raw32"
  [task_time_s] -> Test Detection Criteria1/2
  [VDDM_EPBLockTODet_flg] -> DTC_Info/1
  [VDDM_EPBLockTOCFS_flg] -> DTC_Info/3
  Constant20/1 -> Test Detection Criteria1/3
  Constant2/1 -> Switch6/1
  Constant22/1 -> Test Detection Criteria1/4
  Logical Operator3/1 -> Switch6/3, [VDDM_EPBLockTOTestFail_flg]
  [VDDM_EPBLockTOPass_flg] -> DTC_Info/2
  Switch6/1 -> Test Detection Criteria1/1
  [VDDM_EPBLockTOCFS_flg] -> VDDM_EPBLockTOCFS_flg/1
  [VDDM_EPBUnlockTOCFS_flg] -> VDDM_EPBUnlockTOCFS_flg/1
  VDDM_EPB1RCErr_flg/1 -> [VDDM_EPB1RCErr_flg]
  VDDM_EPB1NoCom_flg/1 -> [VDDM_EPB1NoCom_flg]
  VDDM_EPB1CSErr_flg/1 -> [VDDM_EPB1CSErr_flg]
  Equal40/1 -> [VDDM_EPB1RCErrPass_flg]  "VDDM_EPB1RCErrPass_flg"
  [VDDM_EPB1CSErrCFS_flg] -> Delay2/1
  NOT3/1 -> Logical Operator71/2
  Constant77/1 -> Equal42/2
  Equal37/1 -> Logical Operator65/1
  Constant84/1 -> Equal45/2
  [VDDM_EPB1RCErrCFSRls_flg] -> Switch2/2
  Equal36/1 -> [VDDM_EPB1CSErrPass_flg]  "VDDM_EPB1CSErrPass_flg"
  [VDDM_EPB1RCErr_flg] -> Logical Operator69/3
  Relational Operator2/1 -> Terminator1/1  "VDDM_EPB1NoComDFS_flg"
  [DTC_clear_request] -> DTC_Info2/4
  [VDDM_EPB1NoComCFS_flg] -> Logical Operator56/1
  Logical Operator56/1 -> Logical Operator67/4
  Constant78/1 -> Timer5/4
  Logical Operator70/1 -> Logical Operator52/3
  Delay1/1 -> NOT1/1
  Constant60/1 -> Logical Operator52/4
  [DTC_clear_request] -> Logical Operator52/2
  NOT1/1 -> Logical Operator70/2
  Logical Operator10/1 -> Logical Operator52/1
  Constant71/1 -> Equal41/2
  Logical Operator67/1 -> Timer5/1, Logical Operator64/1
  Test Detection Criteria5/1 -> [VDDM_EPB1CSErrDet_flg]  "VDDM_EPB1CSErrDet_flg"
  [task_time_s] -> Test Detection Criteria5/2
  [VDDM_EPB1NoComCFS_flg] -> Logical Operator53/1
  [VDDM_EPB1CSErrDet_flg] -> DTC_Info4/1
  Test Detection Criteria3/1 -> [VDDM_EPB1NoComDet_flg]  "VDDM_EPB1NoComDet_flg"
  [DTC_clear_request] -> DTC_Info3/4
  [DTC_clear_request] -> DTC_Info4/4
  Switch4/1 -> Test Detection Criteria3/1
  Test Detection Criteria4/1 -> [VDDM_EPB1RCErrDet_flg]  "VDDM_EPB1RCErrDet_flg"
  DTC_Couter4/1 -> [VDDM_EPB1CSErrCFS_flg]  "VDDM_EPB1CSErrCFS_flg"
  Logical Operator13/1 -> Logical Operator58/1
  [VDDM_EPB1NoComCFS_flg] -> Delay1/1
  DTC_Couter3/1 -> [VDDM_EPB1NoComCFS_flg]  "VDDM_EPB1NoComCFS_flg"
  Logical Operator58/1 -> [VDDM_EPB1RCErrCFSRls_flg]  "VDDM_EPB1RCErrCFSRls_flg"
  [VDDM_EPB1NoComPass_flg] -> Logical Operator70/1
  Relational Operator1/1 -> Terminator5/1  "VDDM_EPB1CSErrDFS_flg"
  [VDDM_EPB1CSErrCFSRls_flg] -> Switch3/2
  [VDDM_EPB1RCErrCFSRls_flg] -> DTC_Couter7/2
  [VDDM_EPB1CSErrDet_flg] -> DTC_Couter4/1
  [VPMM_SysPwrSta_enum] -> Equal45/1
  Equal39/1 -> [VDDM_EPB1NoComPass_flg]  "VDDM_EPB1NoComPass_flg"
  [VDDM_EPB1CSErrCFSRls_flg] -> DTC_Couter4/2
  Logical Operator52/1 -> [VDDM_EPB1NoComCFSRls_flg]  "VDDM_EPB1NoComCFSRls_flg"
  Constant102/1 -> Relational Operator3/2
  Switch3/1 -> Test Detection Criteria5/1
  Constant101/1 -> Logical Operator58/4
  [DTC_clear_request] -> Logical Operator58/2
  Logical Operator71/1 -> Logical Operator58/3
  DTC_Couter7/2 -> Relational Operator3/1  "VDDM_EPB1RCErrDTC_cnt"
  Equal38/1 -> Logical Operator72/1
  Constant76/1 -> Relational Operator2/2
  Logical Operator74/1 -> [VDDM_EPB1CSErrCFSRls_flg]  "VDDM_EPB1CSErrCFSRls_flg"
  Constant62/1 -> DTC_Couter3/3
  NOT2/1 -> Logical Operator76/2
  [VPMM_SysPwrSta_enum] -> Equal38/1
  Equal41/1 -> Logical Operator69/1
  [VPMM_SysPwrSta_enum] -> Equal37/1
  Constant81/1 -> Equal37/2
  Constant24/1 -> DTC_Couter7/3
  [VDDM_EPB1RCErrDet_flg] -> DTC_Couter7/1
  Logical Operator53/1 -> Logical Operator60/4
  DTC_Couter7/1 -> [VDDM_EPB1RCErrCFS_flg]  "VDDM_EPB1RCErrCFS_flg"
  [VPMM_SysPwrSta_enum] -> Equal42/1
  DTC_Couter3/2 -> Relational Operator2/1  "VDDM_EPB1NoComDTC_cnt"
  [VDDM_EPB1NoCom_flg] -> Logical Operator73/1
  Constant83/1 -> Equal29/2
  [VPMM_SysPwrSta_enum] -> Equal29/1
  Equal45/1 -> Logical Operator67/1
  Constant59/1 -> DTC_Couter4/3
  Constant74/1 -> Equal36/2
  Logical Operator66/1 -> Logical Operator63/4
  [task_time_s] -> Test Detection Criteria4/2
  [task_time_s] -> Timer4/3
  Constant65/1 -> Switch4/1
  Logical Operator69/1 -> Switch2/3
  Constant56/1 -> Test Detection Criteria4/3
  [VDDM_EPB1CSErr_flg] -> Logical Operator63/3
  Equal42/1 -> Logical Operator60/1
  Logical Operator57/1 -> Timer4/2
  DTC_Info2/1 -> VDDM_EPB1NoComDTC_raw32/1  "VDDM_EPB1NoComDTC_raw32"
  Delay3/1 -> NOT3/1
  Logical Operator73/1 -> Logical Operator72/3
  Constant67/1 -> Equal39/2
  [VDDM_EPB1NoComCFSRls_flg] -> Switch4/2
  [VDDM_EPB1RCErrDet_flg] -> DTC_Info3/1
  Logical Operator65/1 -> Switch4/3
  Constant73/1 -> Test Detection Criteria5/3
  Logical Operator63/1 -> Switch3/3
  [VPMM_SysPwrSta_enum] -> Equal41/1
  [task_time_s] -> Test Detection Criteria3/2
  Logical Operator68/1 -> Logical Operator67/3
  Constant57/1 -> Equal40/2
  [VDDM_EPB1NoComCFS_flg] -> Logical Operator66/1
  Switch2/1 -> Test Detection Criteria4/1
  [VDDM_EPB1CSErrPass_flg] -> DTC_Info4/2
  [NO_CAN1_BUS_OFF] -> Logical Operator67/2
  [task_time_s] -> Timer5/3
  Logical Operator64/1 -> Timer5/2
  [VDDM_EPB1CSErr_flg] -> Logical Operator68/1
  Constant64/1 -> Test Detection Criteria4/4
  [VDDM_EPB1RCErrCFS_flg] -> DTC_Info3/3
  [VDDM_EPB1RCErrCFS_flg] -> Delay3/1
  [task_time_s] -> Timer1/3
  [NO_CAN1_BUS_OFF] -> Logical Operator60/2
  [VDDM_EPB1RCErrPass_flg] -> DTC_Info3/2
  Constant70/1 -> Timer1/4
  [NO_CAN1_BUS_OFF] -> Logical Operator69/2
  Timer1/1 -> Equal40/1
  Logical Operator72/1 -> Logical Operator57/1, Timer4/1
  [VDDM_EPB1RCErr_flg] -> Logical Operator62/1
  [NO_CAN1_BUS_OFF] -> Logical Operator65/2
  Constant55/1 -> Switch2/1
  Logical Operator54/1 -> Timer1/2
  [NO_CAN1_BUS_OFF] -> Logical Operator63/2
  Constant72/1 -> Switch3/1
  Constant79/1 -> Timer4/4
  [VDDM_EPB1NoCom_flg] -> Logical Operator65/3
  Constant69/1 -> Test Detection Criteria3/4
  Logical Operator60/1 -> Timer1/1, Logical Operator54/1
  [VDDM_EPB1NoComDet_flg] -> DTC_Info2/1
  [VDDM_EPB1NoComDet_flg] -> DTC_Couter3/1
  DTC_Info3/1 -> VDDM_EPB1RCErrDTC_raw32/1  "VDDM_EPB1RCErrDTC_raw32"
  Delay2/1 -> NOT2/1
  Relational Operator3/1 -> Terminator3/1  "VDDM_EPB1RCErrDFS_flg"
  Constant75/1 -> Test Detection Criteria5/4
  [VDDM_EPB1NoComCFS_flg] -> DTC_Info2/3
  [VDDM_EPB1NoComPass_flg] -> DTC_Info2/2
  [NO_CAN1_BUS_OFF] -> Logical Operator72/2
  Constant37/1 -> Equal38/2
  [VDDM_EPB1RCErrPass_flg] -> Logical Operator71/1
  [VDDM_EPB1CSErrPass_flg] -> Logical Operator76/1
  DTC_Info4/1 -> VDDM_EPB1CSErrDTC_raw32/1  "VDDM_EPB1CSErrDTC_raw32"
  Timer5/1 -> Equal36/1
  Equal29/1 -> Logical Operator63/1
  Logical Operator18/1 -> Logical Operator74/1
  DTC_Couter4/2 -> Relational Operator1/1  "VDDM_EPB1CSErrDTC_cnt"
  Logical Operator76/1 -> Logical Operator74/3
  Constant66/1 -> Test Detection Criteria3/3
  [VDDM_EPB1CSErrCFS_flg] -> DTC_Info4/3
  [DTC_clear_request] -> Logical Operator74/2
  Timer4/1 -> Equal39/1
  [VDDM_EPB1NoComCFS_flg] -> Logical Operator59/1
  Constant48/1 -> Logical Operator74/4
  Logical Operator62/1 -> Logical Operator60/3
  Constant54/1 -> Relational Operator1/2
  [VDDM_EPB1NoComCFSRls_flg] -> DTC_Couter3/2
  Logical Operator59/1 -> Logical Operator69/4
  Switch5/1 -> Test Detection Criteria6/1
  [VDDM_EPBSigErrDet_flg] -> DTC_Info5/2
  Logical Operator86/1 -> Switch5/3
  Constant98/1 -> Test Detection Criteria6/4
  Constant96/1 -> Switch5/1
  Constant97/1 -> Test Detection Criteria6/3
  [VDDM_EPBSigErrCFS_flg] -> DTC_Info5/3
  [VDDM_EPBSigErrDet_flg] -> DTC_Info5/1
  [task_time_s] -> Test Detection Criteria6/2
  DTC_Info5/1 -> VDDM_EPBSigErrDTC_raw32/1  "VDDM_EPBSigErrDTC_raw32"
  Test Detection Criteria6/1 -> [VDDM_EPBSigErrDet_flg]  "VDDM_EPBSigErrDet_flg"
  [VDDM_EPBSigErrCFSRls_flg] -> Switch5/2
  [DTC_clear_request] -> DTC_Info5/4
  Equal47/1 -> Logical Operator86/5
  [NO_CAN1_BUS_OFF] -> Logical Operator86/1
  [VINP_EPBErrSta_enum] -> Logical Operator86/6
  [VDDM_EPB1CSErrCFS_flg] -> Logical Operator91/1
  Logical Operator91/1 -> Logical Operator86/4
  Logical Operator82/1 -> Logical Operator86/2
  Logical Operator90/1 -> Logical Operator86/3
  [VDDM_EPB1NoComCFS_flg] -> Logical Operator82/1
  [VDDM_EPB1RCErrCFS_flg] -> Logical Operator90/1
  [VPMM_SysPwrSta_enum] -> Equal47/1
  Constant85/1 -> Equal47/2
  DTC_Couter6/2 -> Relational Operator4/1  "VDDM_EPBSigErrDTC_cnt"
  Constant89/1 -> DTC_Couter6/3
  Constant94/1 -> Relational Operator4/2
  Logical Operator79/1 -> [VDDM_EPBSigErrCFSRls_flg]  "VDDM_EPBSigErrCFSRls_flg"
  Logical Operator9/1 -> Logical Operator79/1
  [VDDM_EPBSigErrDet_flg] -> DTC_Couter6/1
  Constant88/1 -> Logical Operator79/4
  Logical Operator80/1 -> Logical Operator79/3
  [DTC_clear_request] -> Logical Operator79/2
  Relational Operator4/1 -> Terminator/1  "VDDM_EPBSigErrDFS_flg"
  DTC_Couter6/1 -> [VDDM_EPBSigErrCFS_flg]  "VDDM_EPBSigErrCFS_flg"
  [VDDM_EPBSigErrCFSRls_flg] -> DTC_Couter6/2
  Constant87/1 -> Equal52/2
  [task_time_s] -> Timer6/3
  Equal52/1 -> [VDDM_EPBSigErrPass_flg]  "VDDM_EPBSigErrPass_flg"
  Timer6/1 -> Equal52/1
  Logical Operator92/1 -> Timer6/1, Logical Operator88/1
  Constant95/1 -> Timer6/4
  Logical Operator88/1 -> Timer6/2
  Logical Operator94/1 -> Logical Operator92/4
  Logical Operator89/1 -> Logical Operator92/2
  Logical Operator93/1 -> Logical Operator92/3
  Constant99/1 -> Equal53/2
  [VDDM_EPB1RCErrCFS_flg] -> Logical Operator93/1
  [VDDM_EPB1NoComCFS_flg] -> Logical Operator89/1
  [NO_CAN1_BUS_OFF] -> Logical Operator92/1
  [VINP_EPBErrSta_enum] -> Logical Operator95/1
  Equal53/1 -> Logical Operator92/5
  [VDDM_EPB1CSErrCFS_flg] -> Logical Operator94/1
  [VPMM_SysPwrSta_enum] -> Equal53/1
  Logical Operator95/1 -> Logical Operator92/6
  [VTQD_GearActualPosn_enum] -> Equal54/1
  Equal54/1 -> Logical Operator80/2
  Constant86/1 -> Equal54/2
  [VDDM_EPBSigErrPass_flg] -> Logical Operator80/1
  Constant8/1 -> Equal1/2
  [VPMM_SysPwrSta_enum] -> Equal1/1
  Logical Operator1/1 -> [VDDM_EPBLockTOCFSRls_flg]  "VDDM_EPBLockTOCFSRls_flg"
  [VDDM_EPBLockTOCFSRls_flg] -> DTC_Couter5/2
  [VDDM_EPBLockTODet_flg] -> DTC_Couter5/1
  Constant5/1 -> Logical Operator1/4
  [DTC_clear_request] -> Logical Operator1/2
  [VDDM_EPBLockTOPass_flg] -> Logical Operator1/3
  Logical Operator7/1 -> Logical Operator1/1
  DTC_Couter5/2 -> Relational Operator5/1  "VDDM_EPBLockTODTC_cnt"
  Constant12/1 -> DTC_Couter5/3
  Relational Operator5/1 -> Terminator2/1  "VDDM_EPBLockTODFS_flg"
  DTC_Couter5/1 -> [VDDM_EPBLockTOCFS_flg]  "VDDM_EPBLockTOCFS_flg"
  Constant17/1 -> Relational Operator5/2
  [VPMM_SysPwrSta_enum] -> Equal9/1
  Constant1/1 -> Equal9/2
  [VDDM_EPBUnlockTODFSRls_flg] -> DTC_Couter1/2
  Constant21/1 -> Relational Operator6/2
  [DTC_clear_request] -> Logical Operator23/2
  Relational Operator6/1 -> Terminator4/1  "VDDM_EPBUnlockTODFS_flg"
  [VDDM_EPBUnlockTOPass_flg] -> Logical Operator23/3
  DTC_Couter1/1 -> [VDDM_EPBUnlockTOCFS_flg]  "VDDM_EPBUnlockTOCFS_flg"
  Logical Operator17/1 -> Logical Operator23/1
  DTC_Couter1/2 -> Relational Operator6/1  "VDDM_EPBUnlockTODTC_cnt"
  Constant23/1 -> Logical Operator23/4
  [VDDM_EPBUnlockTODet_flg] -> DTC_Couter1/1
  Constant16/1 -> DTC_Couter1/3
  Logical Operator23/1 -> [VDDM_EPBUnlockTODFSRls_flg]  "VDDM_EPBUnlockTODFSRls_flg"
  [VDDM_EPBSigErrCFS_flg] -> VDDM_EPBSigErrCFS_flg/1
  [VDDM_EPB1NoComCFS_flg] -> VDDM_EPB1NoComCFS_flg/1
  [VDDM_EPB1RCErrCFS_flg] -> VDDM_EPB1RCErrCFS_flg/1
  [VDDM_EPB1CSErrCFS_flg] -> VDDM_EPB1CSErrCFS_flg/1
  Constant26/1 -> Equal18/2
  Constant25/1 -> Equal14/2
  [VPMM_SysPwrSta_enum] -> Equal14/1
  Equal18/1 -> Logical Operator9/1
  Unit Delay1/1 -> Equal18/1
  Equal14/1 -> Logical Operator9/2
  [VPMM_SysPwrSta_enum] -> Unit Delay1/1
  Constant28/1 -> Equal16/2
  Constant27/1 -> Equal15/2
  [VPMM_SysPwrSta_enum] -> Equal15/1
  Equal16/1 -> Logical Operator10/1
  Unit Delay6/1 -> Equal16/1
  Equal15/1 -> Logical Operator10/2
  [VPMM_SysPwrSta_enum] -> Unit Delay6/1
  Constant14/1 -> Equal8/2
  Constant13/1 -> Equal6/2
  [VPMM_SysPwrSta_enum] -> Equal6/1
  Equal8/1 -> Logical Operator7/1
  Unit Delay2/1 -> Equal8/1
  Equal6/1 -> Logical Operator7/2
  [VPMM_SysPwrSta_enum] -> Unit Delay2/1
  Constant30/1 -> Equal19/2
  Constant29/1 -> Equal17/2
  [VPMM_SysPwrSta_enum] -> Equal17/1
  Equal19/1 -> Logical Operator13/1
  Unit Delay7/1 -> Equal19/1
  Equal17/1 -> Logical Operator13/2
  [VPMM_SysPwrSta_enum] -> Unit Delay7/1
  Constant19/1 -> Equal13/2
  Constant18/1 -> Equal12/2
  [VPMM_SysPwrSta_enum] -> Equal12/1
  Equal13/1 -> Logical Operator17/1
  Unit Delay5/1 -> Equal13/1
  Equal12/1 -> Logical Operator17/2
  [VPMM_SysPwrSta_enum] -> Unit Delay5/1
  Constant32/1 -> Equal21/2
  Constant31/1 -> Equal20/2
  [VPMM_SysPwrSta_enum] -> Equal20/1
  Equal21/1 -> Logical Operator18/1
  Unit Delay8/1 -> Equal21/1
  Equal20/1 -> Logical Operator18/2
  [VPMM_SysPwrSta_enum] -> Unit Delay8/1
  [VINP_ShifterHandleCmd_enum] -> Terminator6/1
  Constant51/1 -> Equal3/2
  [VDDM_EPBUnlockTOCFS_flg] -> Logical Operator34/1
  Logical Operator34/1 -> Logical Operator31/6
  Equal4/1 -> AND1/2
  [VDDM_EPB1CSErrCFS_flg] -> Logical Operator39/1
  [NO_CAN1_BUS_OFF] -> Logical Operator31/1
  Logical Operator5/1 -> Logical Operator31/2
  [VPMM_SysPwrSta_enum] -> Equal3/1
  SR_Latch1/1 -> [VDDM_EPBLockTOPass_flg]  "VDDM_EPBLockTOPass_flg"
  [VDDM_EPB1RCErrCFS_flg] -> Logical Operator38/1
  Logical Operator31/1 -> SR_Latch1/1
  Logical Operator38/1 -> Logical Operator31/3
  AND1/1 -> AND4/1
  [VDDM_EPB1NoComCFS_flg] -> Logical Operator5/1
  Constant10/1 -> Equal4/2
  [VTQD_ActParkRequest_flg] -> AND1/1
  SR_Latch/1 -> Logical Operator20/1, Timer7/1, AND4/2
  [VTQD_ActParkRequest_flg] -> Detect Increase/1
  Constant33/1 -> Timer7/4
  Delay/1 -> SR_Latch/2
  Detect Increase/1 -> SR_Latch/1
  AND4/1 -> Logical Operator31/7
  [VDDM_EPBLockTOTestFail_flg] -> SR_Latch1/2
  Logical Operator39/1 -> Logical Operator31/4
  Logical Operator20/1 -> Timer7/2
  Timer7/1 -> Equal22/1
  Equal22/1 -> Delay/1
  [VINP_EPBSta_enum] -> Equal4/1
  Constant34/1 -> Equal22/2
  [task_time_s] -> Timer7/3
  Equal3/1 -> Logical Operator31/5
  Logical Operator11/1 -> Logical Operator2/2
  Logical Operator15/1 -> Logical Operator2/3
  Logical Operator14/1 -> Timer2/2
  [VDDM_EPB1NoComCFS_flg] -> Logical Operator11/1
  [VINP_EPBSta_enum] -> Equal10/1
  Constant4/1 -> Equal11/2
  Unit Delay4/1 -> Logical Operator6/1
  Constant6/1 -> Equal7/2
  Timer2/1 -> Equal7/1
  Logical Operator6/1 -> Logical Operator2/6
  Constant15/1 -> Timer2/4
  Logical Operator8/1 -> AND3/1
  [VDDM_EPBUnlockTOTestFail_flg] -> SR_Latch3/2
  Equal7/1 -> Delay4/1
  [VPMM_SysPwrSta_enum] -> Equal11/1
  [VDDM_EPB1CSErrCFS_flg] -> Logical Operator16/1
  [NO_CAN1_BUS_OFF] -> Logical Operator2/1
  Delay4/1 -> SR_Latch2/2
  Detect Decrease/1 -> SR_Latch2/1
  [VTQD_ActParkRequest_flg] -> Detect Decrease/1
  [VDDM_EPBLockTOCFS_flg] -> Unit Delay4/1
  Equal11/1 -> Logical Operator2/5
  AND3/1 -> AND5/1
  SR_Latch3/1 -> [VDDM_EPBUnlockTOPass_flg]  "VDDM_EPBUnlockTOPass_flg"
  SR_Latch2/1 -> Logical Operator14/1, AND5/2, Timer2/1
  Logical Operator2/1 -> SR_Latch3/1
  AND5/1 -> Logical Operator2/7
  [VDDM_EPB1RCErrCFS_flg] -> Logical Operator15/1
  Logical Operator16/1 -> Logical Operator2/4
  [VTQD_ActParkRequest_flg] -> Logical Operator8/1
  [task_time_s] -> Timer2/3
  Constant7/1 -> Equal10/2
  Equal10/1 -> AND3/2
  [VDDM_EPB1NoComCFS_flg] -> Logical Operator/1
  [VDDM_EPB1RCErrCFS_flg] -> Logical Operator/2
  [VDDM_EPB1CSErrCFS_flg] -> Logical Operator/3
  Logical Operator/1 -> VDDM_EPB1Err_flg/1  "VDDM_EPB1Err_flg"
  SR_Latch4/1 -> Logical Operator19/7
  [VTQD_ActParkRequest_flg] -> Detect Decrease1/1
  Detect Decrease1/1 -> AND2/1
  AND2/1 -> SR_Latch4/1
  Constant3/1 -> Equal2/2
  Equal2/1 -> SR_Latch4/2
  [VINP_EPBSta_enum] -> Equal2/1
